simulink library "Chassis_Axle1"  (R2026a)
settings: Solver=VariableStepAuto
undefined symbols (not defined in the file): Init, Vehicle
libraries: Tire_1x2x x2, Aero_Coefficients x1, Body_Axle1 x1, Dampers_Axle1 x1, Springs_Axle1 x1, Suspension x1
Description:
  | Component of Simscape Vehicle Templates Library
  | 
  | Copyright 2018-2026 The MathWorks, Inc.
settings Model: Creator=smiller  LastModifiedBy=smiller

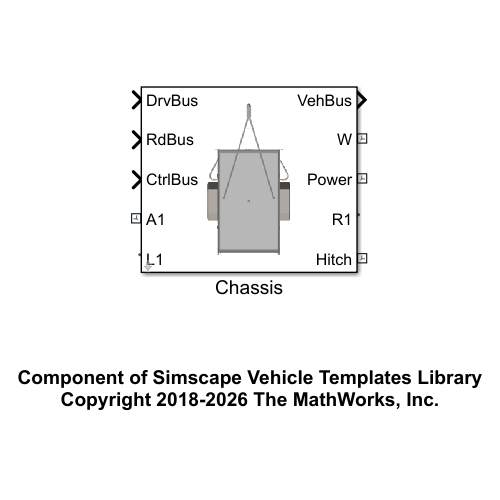
[thumbnail: Simulink's stored preview of the top-level diagram]
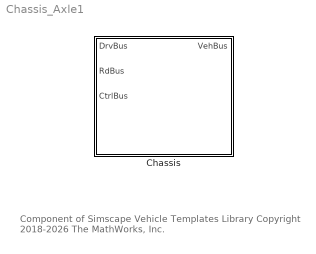
== system Chassis_Axle1 ==
  note: Component of Simscape Vehicle Templates Library
      | Copyright 2018-2026 The MathWorks, Inc.
  Chassis : Subsystem  Tag=PublishSubsystem  VariantControl=Chassis  mask(Chassis){Chassis=Vehicle.Chassis, Init=Init, veh_index=61}
      mask prompts: Chassis "Vehicle Parameters"; Init "Initial Values"; veh_index "Vehicle Index (for tires)"
      mask help: Models vehicle chassis, with suspension, body, tires, springs, and dampers.
      mask Help: web('sm_car_doc_chassis.html')
      mask Display:
      | % Get image from BodyGeometry.class
      | % (active choice for Body Geometry subsystem)
      | temp_veh_bg_class = lower(get_param([gcb '/Body/Body Geometry'],'LabelModeActiveChoice'));
      | 
      | imagestr = (['sm_car_chassis_' temp_veh_bg_class '.png']);
      | if(~exist(imagestr))
      |     imagestr = ['sm_car_chassis_default.png'];
      | end
      | 
      | image(imagestr);

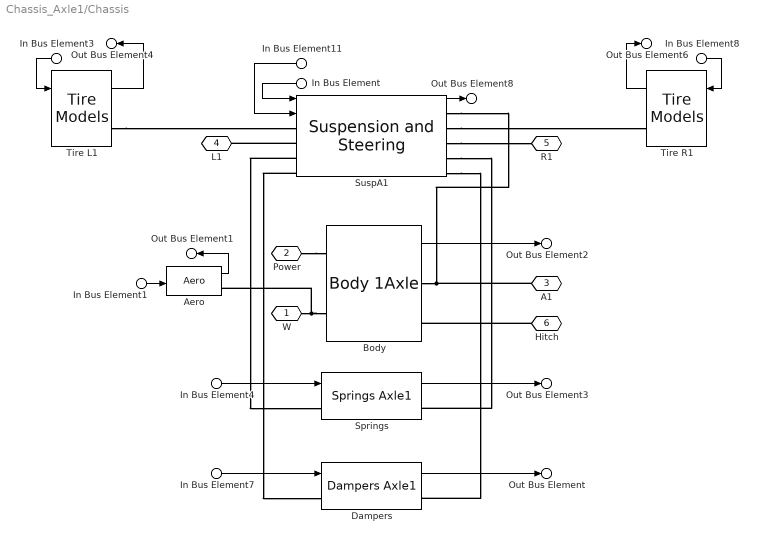
== system Chassis_Axle1/Chassis ==
  In Bus Element11 : Inport  PortName=DrvBus
  In Bus Element3 : Inport  Port=2  PortName=RdBus  Element=L1
  In Bus Element8 : Inport  Port=2  PortName=RdBus  Element=R1
  In Bus Element1 : Inport  Port=2  PortName=RdBus  Element=fWindTrailer
  In Bus Element7 : Inport  Port=3  PortName=CtrlBus  Element=Damper
  In Bus Element : Inport  Port=3  PortName=CtrlBus  Element=SuspA1
  In Bus Element4 : Inport  Port=3  PortName=CtrlBus  Element=Spring
  Aero : Aero_Coefficients/Aero  CL=Chassis.Aero.CL.Value  CD=Chassis.Aero.CD.Value  rho=Chassis.Aero.rho_air.Value  A=Chassis.Aero.ARef.Value  sCentreOfPressure=Chassis.Aero.sPressureCentre.Value  clr_hp=Visual.hp.clr  opc_hp=Visual.hp.opc  rad_hp=Visual.hp.rad
  Body : Body_Axle1/Body 1Axle  hp_mount_fa=Chassis.Body.sAxle1.Value  hp_mount_hitch=Chassis.Body.sHitch.Value  hp_mount_power=Chassis.Body.sPower.Value  hp_chassis_cg=Chassis.Body.sCG.Value  chassis_mass=Chassis.Body.m.Value  chassis_inertia=Chassis.Body.J.Value  clr_chassis_hp_cg=Visual.hp.clr  opc_chassis_hp_cg=Visual.hp.opc  size_chassis_hp_cg=Visual.hp.rad  BodyGeometry=Chassis.Body.BodyGeometry
  Dampers : Dampers_Axle1/Dampers Axle1  VariantControl=Variant1  LabelModeActiveChoice=Independent  Damper=Vehicle.Chassis.Damper  VariantLabel=Vehicle.Chassis.Damper.class.Value
      settings: AttributesFormatString=%<ActiveVariant>
  Springs : Springs_Axle1/Springs Axle1  VariantControl=Variant1  LabelModeActiveChoice=Independent  Spring=Vehicle.Chassis.Spring  VariantLabel=Vehicle.Chassis.Spring.class.Value
      settings: AttributesFormatString=%<ActiveVariant>
  SuspA1 : Suspension/Suspension and Steering  VariantControl=Variant1  LabelModeActiveChoice=Linkage  Susp=Chassis.SuspA1  Init=Init.Axle1  VariantLabel=Chassis.SuspA1.class.Value
      settings: AttributesFormatString=%<LabelModeActiveChoice>
  Tire L1 : Tire_1x2x/Tire Models  Tag=PublishSubsystem  VariantControl=Variant1  LabelModeActiveChoice=MFMbody  popup_leftRight=Left  tir_index=veh_index  Tire=Chassis.TireA1  VariantLabel=Chassis.TireA1.class.Value
      settings: AttributesFormatString=%<ActiveVariant>
  Tire R1 : Tire_1x2x/Tire Models  Tag=PublishSubsystem  VariantControl=Variant1  LabelModeActiveChoice=MFMbody  popup_leftRight=Right  tir_index=veh_index+4  Tire=Chassis.TireA1  VariantLabel=Chassis.TireA1.class.Value
      settings: AttributesFormatString=%<ActiveVariant>
  W : PMIOPort  Side=Right
  Power : PMIOPort  Port=2  Side=Right
  A1 : PMIOPort  Port=3  Side=Left
  L1 : PMIOPort  Port=4  Side=Left
  R1 : PMIOPort  Port=5  Side=Right
  Hitch : PMIOPort  Port=6  Side=Right
  Out Bus Element4 : Outport  VectorParamsAs1DForOutWhenUnconnected=off  PortName=VehBus  Element=WhlL1
  Out Bus Element6 : Outport  VectorParamsAs1DForOutWhenUnconnected=off  PortName=VehBus  Element=WhlR1
  Out Bus Element1 : Outport  VectorParamsAs1DForOutWhenUnconnected=off  PortName=VehBus  Element=Aero
  Out Bus Element : Outport  VectorParamsAs1DForOutWhenUnconnected=off  PortName=VehBus  Element=Damper
  Out Bus Element3 : Outport  VectorParamsAs1DForOutWhenUnconnected=off  PortName=VehBus  Element=Spring
  Out Bus Element8 : Outport  VectorParamsAs1DForOutWhenUnconnected=off  PortName=VehBus  Element=SuspA1
  Out Bus Element2 : Outport  VectorParamsAs1DForOutWhenUnconnected=off  PortName=VehBus  Element=Body
  wires:
  Springs/1 -> Out Bus Element3/1
  Dampers/1 -> Out Bus Element/1
  In Bus Element3/1 -> Tire L1/1
  Tire R1/1 -> Out Bus Element6/1
  In Bus Element8/1 -> Tire R1/1
  Tire L1/1 -> Out Bus Element4/1
  In Bus Element11/1 -> SuspA1/2
  SuspA1/1 -> Out Bus Element8/1
  In Bus Element/1 -> SuspA1/1
  In Bus Element7/1 -> Dampers/1
  In Bus Element4/1 -> Springs/1
  Aero/1 -> Out Bus Element1/1
  In Bus Element1/1 -> Aero/1
  Body/1 -> Out Bus Element2/1
  connections:
  W/RConn1 -- Aero/RConn1 -- Body/LConn2
  SuspA1/LConn2 -- L1/RConn1
  SuspA1/RConn3 -- R1/RConn1
  SuspA1/RConn2 -- Tire R1/RConn1
  Tire L1/RConn1 -- SuspA1/LConn1
  A1/RConn1 -- SuspA1/RConn1 -- Body/RConn1
  SuspA1/LConn3 -- Springs/LConn1
  SuspA1/RConn4 -- Springs/RConn1
  SuspA1/LConn4 -- Dampers/LConn1
  SuspA1/RConn5 -- Dampers/RConn1
  Hitch/RConn1 -- Body/RConn2
  Power/RConn1 -- Body/LConn1
